simulink subsystem "hyper_saturation"  (R2022a)
settings: Solver=VariableStepAuto  StartTime=0.0  StopTime=10.0  RelTol=1e-3
settings Model: Creator=Niccolò  LastModifiedBy=Niccolò

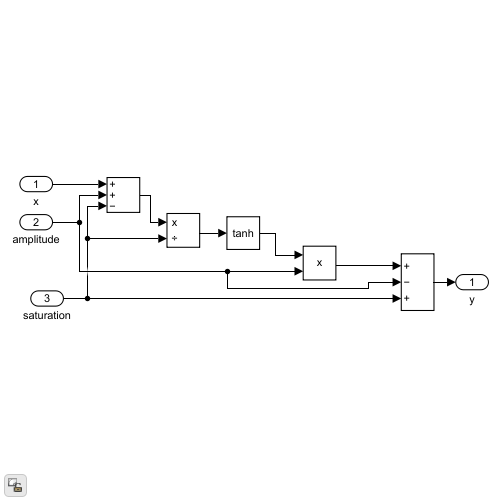
[thumbnail: Simulink's stored preview of the top-level diagram]
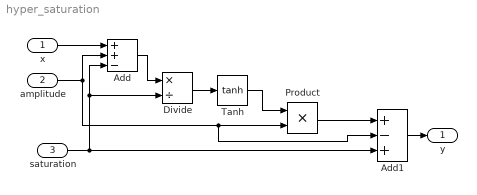
== system hyper_saturation ==
  x : Inport
  amplitude : Inport  Port=2
  saturation : Inport  Port=3
  Add : Sum  Inputs=++-
  Add1 : Sum  Inputs=+-+
  Divide : Product  Inputs=*/
  Product : Product
  Tanh : Trigonometry  Operator=tanh
  y : Outport
  wires:
  saturation/1 -> Add/3, Divide/2, Add1/3
  Add/1 -> Divide/1
  Tanh/1 -> Product/1
  amplitude/1 -> Add/2, Product/2, Add1/2
  Add1/1 -> y/1
  Product/1 -> Add1/1
  Divide/1 -> Tanh/1
  x/1 -> Add/1
